simulink model "Multi_Scenario_WECS_based_Microgrid_2017"  (R2025a)
settings: Solver=ode45  StartTime=0.0  StopTime=4  RelTol=1e-3  EnableMultiTasking=on
undefined symbols (not defined in the file): c1, c2, c3, c4, c5, c6, DiscIntNeverNeededParam, fdesignblkfcn, gcbh, Hydride, Metal, Nickel
libraries: powerlib x63, powerlib_extras x26, powerlib_meascontrol x25, simulink x5, simulink_extras x2, electricdrivelib x1
(part 4 of 4)

== system Multi_Scenario_WECS_based_Microgrid_2017/Generator side control1/Discrete SV PWM Generator/SV Modulator Pattern #1/Generate pulse pattern/Determine interval of the PWM period based on Ta Tb and To ==
  TaTbTo : Inport
  Constant7 : Constant
  Demux1 : Demux  Outputs=6
      settings: DisplayOption=none
  Relational Operator{,1..5} (6 alike) : RelationalOperator  InputSameDT=off
  Subsystem : Subsystem
  Sum1 : Sum  Inputs=+++++++  SaturateOnIntegerOverflow=on
  Triangle : simulink/Sources/Repeating Sequence  rep_seq_t=[0 1/Fc]  rep_seq_y=[0 1/Fc]
  Tn : Outport
  wires:
  Sum1/1 -> Tn/1
  Demux1/6 -> Relational Operator4/2
  Demux1/5 -> Relational Operator3/2
  Demux1/4 -> Relational Operator2/2
  Demux1/3 -> Relational Operator1/2
  Demux1/2 -> Relational Operator/2
  Demux1/1 -> Relational Operator5/2
  Constant7/1 -> Sum1/1
  Relational Operator5/1 -> Sum1/2
  Relational Operator/1 -> Sum1/3
  Relational Operator1/1 -> Sum1/4
  Relational Operator2/1 -> Sum1/5
  Relational Operator3/1 -> Sum1/6
  Relational Operator4/1 -> Sum1/7
  Triangle/1 -> Relational Operator5/1, Relational Operator/1, Relational Operator1/1, Relational Operator2/1, Relational Operator3/1, Relational Operator4/1
  Subsystem/1(Timing) -> Demux1/1
  TaTbTo/1 -> Subsystem/1(TaTbTo)

== system Multi_Scenario_WECS_based_Microgrid_2017/Generator side control1/Discrete SV PWM Generator/SV Modulator Pattern #1/Generate pulse pattern/Determine interval of the PWM period based on Ta Tb and To/Subsystem ==
  TaTbTo : Inport
  "  1/2" : Gain  Gain=0.5  SaturateOnIntegerOverflow=on  OutDataTypeStr=Inherit: Same as input  ParamDataTypeStr=Inherit: Same as input
  " 1/2" : Gain  Gain=0.5  SaturateOnIntegerOverflow=on  OutDataTypeStr=Inherit: Same as input  ParamDataTypeStr=Inherit: Same as input
  " 1/2 " : Gain  Gain=0.5  SaturateOnIntegerOverflow=on  OutDataTypeStr=Inherit: Same as input  ParamDataTypeStr=Inherit: Same as input
  1/4 : Gain  Gain=0.25  SaturateOnIntegerOverflow=on  OutDataTypeStr=Inherit: Same as input  ParamDataTypeStr=Inherit: Same as input
  Demux : Demux  Outputs=3
      settings: DisplayOption=none
  Mux1 : Mux  Inputs=6
  Sum{5..9} (5 alike) : Sum  SaturateOnIntegerOverflow=on
  Timing : Outport
  wires:
  Mux1/1 -> Timing/1
  Sum5/1 -> Mux1/2, Sum6/1
  Sum6/1 -> Mux1/3, Sum7/1
  Sum7/1 -> Mux1/4, Sum8/1
  Sum8/1 -> Mux1/5, Sum9/1
  Sum9/1 -> Mux1/6
  1/4/1 -> Mux1/1, Sum5/1
  Demux/1 -> " 1/2 "/1
  Demux/2 -> "  1/2"/1
  " 1/2"/1 -> Sum7/2
  TaTbTo/1 -> Demux/1
  "  1/2"/1 -> Sum6/2, Sum8/2
  Demux/3 -> 1/4/1, " 1/2"/1
  " 1/2 "/1 -> Sum5/2, Sum9/2
